simulink model "FinalProjectSim"  (R2022a)
settings: Solver=VariableStepAuto  StartTime=0.0  StopTime=10.0  RelTol=1e-3
values from neighbouring files (symbols this model uses):
  CL_0 = 0.307    [FinalProject.m]
  CL_a = 4.41    [FinalProject.m]
  CL_DM = 0    [FinalProject.m]
  CL_el = 0.43    [FinalProject.m]
  CM_0 = 0.04    [FinalProject.m]
  CM_a = -0.613    [FinalProject.m]
  CM_el = -1.122    [FinalProject.m]
  el = 0.0278    [FinalProject.m]
  k = 0.0554    [FinalProject.m]
  rho = 2.377e-3    (= 0.002377)    [FinalProject.m]
  S = 174    [FinalProject.m]
  W = 2650    [FinalProject.m]
undefined symbols (not defined in the file or in its folder): CD_M
settings Model: Creator=nickmondora  LastModifiedBy=nickmondora

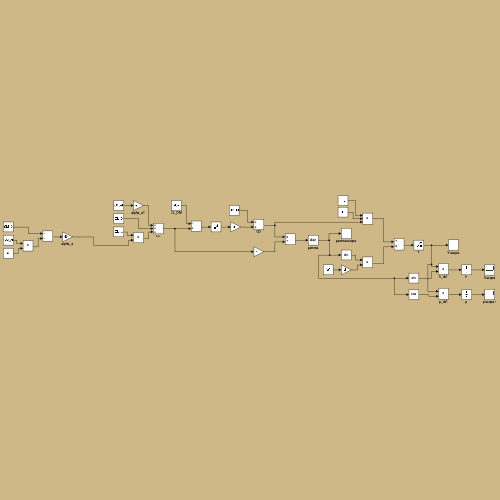
[thumbnail: Simulink's stored preview of the top-level diagram]
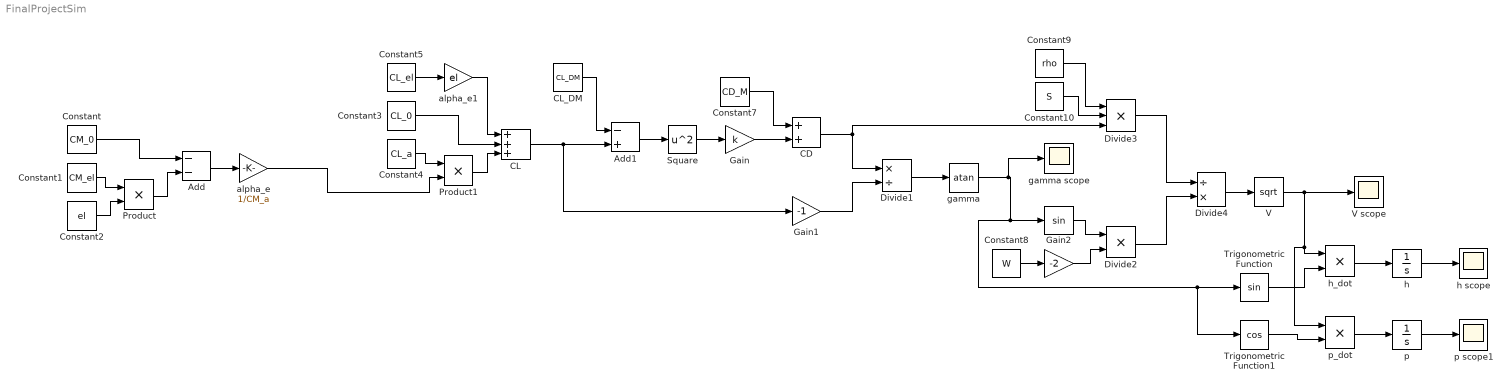
== system FinalProjectSim ==
  " " : Trigonometry
  Add : Sum  Inputs=--
  Add1 : Sum  Inputs=-+
  CD : Sum
  CL : Sum  Inputs=+++
  CL_DM : Constant  Value=CL_DM
  Constant : Constant  Value=CM_0
  Constant1 : Constant  Value=CM_el
  Constant10 : Constant  Value=S
  Constant2 : Constant  Value=el
  Constant3 : Constant  Value=CL_0
  Constant4 : Constant  Value=CL_a
  Constant5 : Constant  Value=CL_el
  Constant7 : Constant  Value=CD_M
  Constant8 : Constant  Value=W
  Constant9 : Constant  Value=rho
  Divide1 : Product  Inputs=*/
  Divide2 : Product  Inputs=**
  Divide3 : Product  Inputs=***
  Divide4 : Product  Inputs=/*
  Gain : Gain  Gain=k
  Gain1 : Gain  Gain=-1
  Gain2 : Gain  Gain=-2
  Product : Product
  Product1 : Product
  Square : Math  Operator=square  SignedPower=on  RndMeth=Zero
  Trigonometric Function : Trigonometry
  Trigonometric Function1 : Trigonometry  Operator=cos
  V : Sqrt
  V scope : Scope
  alpha_e : Gain  Gain=1/CM_a
  alpha_e1 : Gain  Gain=el
  gamma : Trigonometry  Operator=atan
  gamma scope : Scope
  h : Integrator
  h scope : Scope
  h_dot : Product  Inputs=**
  p : Integrator
  p scope1 : Scope
  p_dot : Product  Inputs=**
  wires:
  Constant1/1 -> Product/1
  Constant2/1 -> Product/2
  Constant/1 -> Add/1
  Product/1 -> Add/2
  Add/1 -> alpha_e/1
  Constant3/1 -> CL/2
  Constant4/1 -> Product1/1
  Product1/1 -> CL/3
  alpha_e/1 -> Product1/2
  CL_DM/1 -> Add1/1
  Add1/1 -> Square/1
  Square/1 -> Gain/1
  Gain/1 -> CD/2
  Constant7/1 -> CD/1
  CL/1 -> Gain1/1, Add1/2
  CD/1 -> Divide1/1, Divide3/3
  Gain1/1 -> Divide1/2
  Divide1/1 -> gamma/1
  Constant8/1 -> Gain2/1
  gamma/1 -> gamma scope/1, " "/1, Trigonometric Function1/1, Trigonometric Function/1
  " "/1 -> Divide2/1
  Gain2/1 -> Divide2/2
  Constant9/1 -> Divide3/1
  Constant10/1 -> Divide3/2
  Divide3/1 -> Divide4/1
  Divide2/1 -> Divide4/2
  Divide4/1 -> V/1
  Constant5/1 -> alpha_e1/1
  alpha_e1/1 -> CL/1
  V/1 -> V scope/1, h_dot/1, p_dot/1
  Trigonometric Function/1 -> h_dot/2
  h_dot/1 -> h/1
  h/1 -> h scope/1
  Trigonometric Function1/1 -> p_dot/2
  p_dot/1 -> p/1
  p/1 -> p scope1/1
